simulink model "Introduction_to_Simulink"  (R2015a)
settings: Solver=ode45  StartTime=0.0  StopTime=30  MaxStep=0.1  RelTol=1e-3
undefined symbols (not defined in the file): F, F_n, k, m
settings Model: Creator=tlantela  LastModifiedBy=tlantela

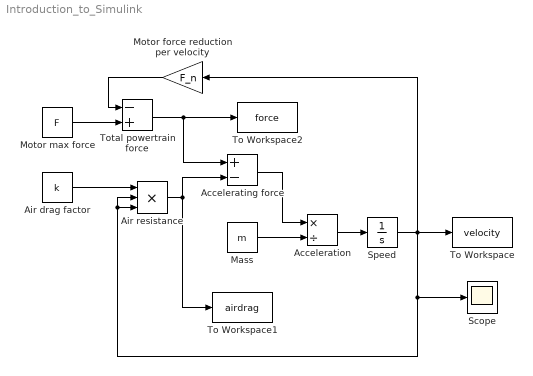
== system Introduction_to_Simulink ==
  Accelerating force : Sum  Inputs=+-
  Acceleration : Product  Inputs=*/
  Air drag factor : Constant  Value=k
  Air resistance : Product  Inputs=3
  Mass : Constant  Value=m
  Motor force reduction per velocity : Gain  Gain=F_n
  Motor max force : Constant  Value=F
  Scope : Scope
  Speed : Integrator
  To Workspace : ToWorkspace  VariableName=velocity  SaveFormat=Timeseries  SampleTime=-1
  To Workspace1 : ToWorkspace  VariableName=airdrag  SaveFormat=Timeseries  SampleTime=-1
  To Workspace2 : ToWorkspace  VariableName=force  SaveFormat=Timeseries  SampleTime=-1
  Total powertrain force : Sum  Inputs=-+
  wires:
  Mass/1 -> Acceleration/2
  Acceleration/1 -> Speed/1
  Air drag factor/1 -> Air resistance/1
  Speed/1 -> Motor force reduction per velocity/1, Scope/1, Air resistance/2, Air resistance/3, To Workspace/1
  Air resistance/1 -> To Workspace1/1, Accelerating force/2
  Accelerating force/1 -> Acceleration/1
  Total powertrain force/1 -> Accelerating force/1, To Workspace2/1
  Motor force reduction per velocity/1 -> Total powertrain force/1
  Motor max force/1 -> Total powertrain force/2
